simulink model "HelicopterLinear"  (R2023a)
settings: Solver=ode4  StartTime=0.0  StopTime=inf  FixedStep=0.1  RelTol=1e-3
values from neighbouring files (symbols this model uses):
  A_c = [0, 0, 1, 0 ... (first row only)    [init.m]
  B_c = [0, 0 ... (first row only)    [init.m]
  B_p = 0.01    [init.m]
  B_y = 0.08    [init.m]
  g = 9.81    [init.m]
  j_eq_p = 0.0172    [init.m]
  j_eq_y = 0.0210    (= 0.021)    [init.m]
  K_pp = 0.0556    [init.m]
  K_py = 0.005    [init.m]
  K_yp = 0.15    [init.m]
  K_yy = 0.21084    [init.m]
  l_cm = 0.015    [init.m]
  m_heli = 0.479    [init.m]
  psi_op = pi/2    (= 1.57079632679)    [init.m]
  teta_op = -10*pi/180    (= -0.174532925199)    [init.m]
  V_mp_op = K_yy*m_heli*g*cos(teta_op)*l_cm/(K_yy*K_pp - K_yp*K_py)    [init.m]
  v_my_op = K_yp*V_mp_op/K_yy    [init.m]
  wpsi_op = 0    [init.m]
  wteta_op = 0    [init.m]
libraries: simulink_extras x6
settings Model: Creator=Jardar Fagerlund  LastModifiedBy=Jardar Fagerlund

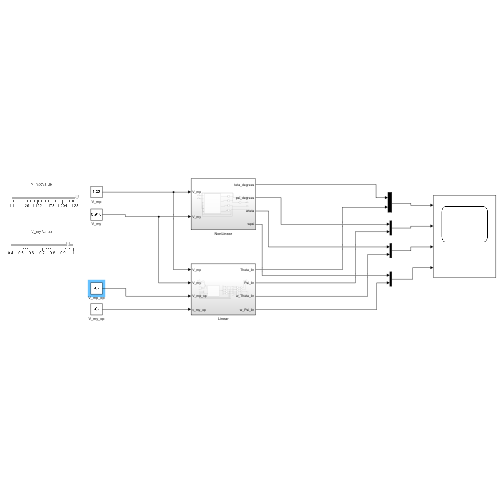
[thumbnail: Simulink's stored preview of the top-level diagram]
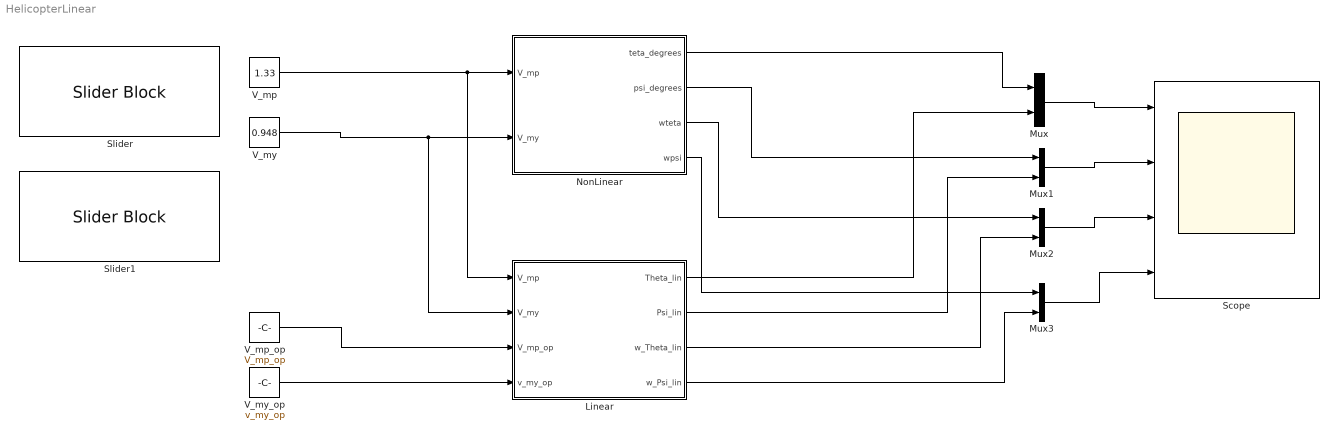
== system HelicopterLinear ==
  Linear : Subsystem
  Mux{,1..3} (4 alike) : Mux  Inputs=2
  NonLinear : Subsystem
  Scope : Scope  NumInputPorts=4
  Slider : SliderBlock  ScaleMin=1.1  ScaleMax=1.23
  Slider1 : SliderBlock  ScaleMin=0.4  ScaleMax=1
  V_mp : Constant  Value=1.33
  V_mp_op : Constant  Value=V_mp_op
  V_my : Constant  Value=0.948
  V_my_op : Constant  Value=v_my_op
  wires:
  V_mp/1 -> Linear/1(V_mp), NonLinear/1(V_mp)
  V_my/1 -> Linear/2(V_my), NonLinear/2(V_my)
  NonLinear/1(teta_degrees) -> Mux/1
  NonLinear/2(psi_degrees) -> Mux1/1
  Linear/1(Theta_lin) -> Mux/2
  Linear/2(Psi_lin) -> Mux1/2
  Mux/1 -> Scope/1
  Mux1/1 -> Scope/2
  Mux2/1 -> Scope/3
  Mux3/1 -> Scope/4
  NonLinear/3(wteta) -> Mux2/1
  Linear/3(w_Theta_lin) -> Mux2/2
  NonLinear/4(wpsi) -> Mux3/1
  Linear/4(w_Psi_lin) -> Mux3/2
  V_mp_op/1 -> Linear/3(V_mp_op)
  V_my_op/1 -> Linear/4(v_my_op)

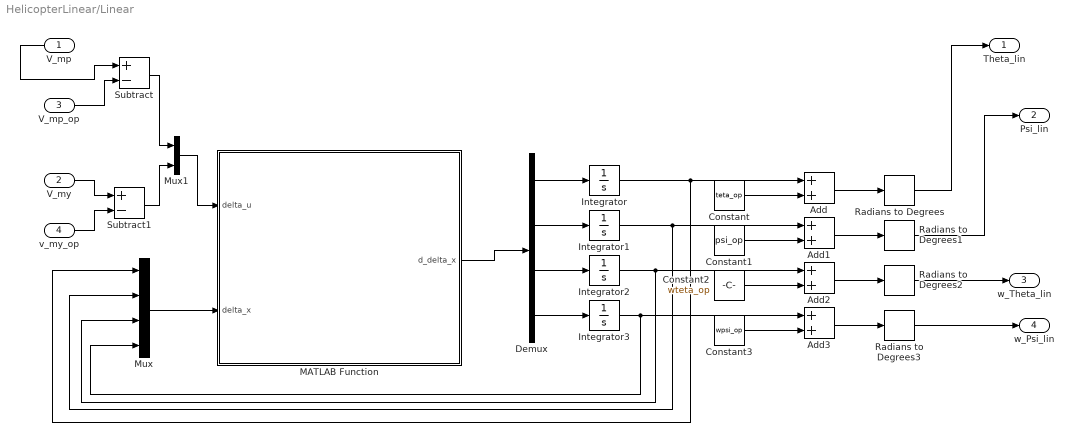
== system HelicopterLinear/Linear ==
  V_mp : Inport
  V_my : Inport  Port=2
  V_mp_op : Inport  Port=3
  v_my_op : Inport  Port=4
  Add{,1..3} (4 alike) : Sum
  Constant : Constant  Value=teta_op
  Constant1 : Constant  Value=psi_op
  Constant2 : Constant  Value=wteta_op
  Constant3 : Constant  Value=wpsi_op
  Demux : Demux
  Integrator : Integrator  LimitOutput=on  UpperSaturationLimit=35*pi/180-teta_op  LowerSaturationLimit=-45*pi/180-teta_op
  Integrator1 : Integrator  LimitOutput=on  UpperSaturationLimit=pi-psi_op  LowerSaturationLimit=0-psi_op
  Integrator2 : Integrator
  Integrator3 : Integrator
  MATLAB Function : MATLAB Function  TreatAsAtomicUnit=on
  Mux : Mux
  Mux1 : Mux  Inputs=2
  Radians to Degrees{,1..3} (4 alike) : simulink_extras/Transformations/Radians to Degrees
  Subtract : Sum  Inputs=+-
  Subtract1 : Sum  Inputs=+-
  Theta_lin : Outport
  Psi_lin : Outport  Port=2
  w_Theta_lin : Outport  Port=3
  w_Psi_lin : Outport  Port=4
  wires:
  Integrator/1 -> Mux/1, Add/1
  Integrator3/1 -> Mux/4, Add3/1
  Integrator1/1 -> Mux/2, Add1/1
  Integrator2/1 -> Mux/3, Add2/1
  Demux/1 -> Integrator/1
  Radians to Degrees1/1 -> Psi_lin/1
  Constant/1 -> Add/2
  Add2/1 -> Radians to Degrees2/1
  Demux/3 -> Integrator2/1
  Demux/4 -> Integrator3/1
  Demux/2 -> Integrator1/1
  Radians to Degrees2/1 -> w_Theta_lin/1
  MATLAB Function/1(d_delta_x) -> Demux/1
  Add3/1 -> Radians to Degrees3/1
  Constant3/1 -> Add3/2
  Constant1/1 -> Add1/2
  Constant2/1 -> Add2/2
  Add/1 -> Radians to Degrees/1
  Add1/1 -> Radians to Degrees1/1
  Radians to Degrees3/1 -> w_Psi_lin/1
  Radians to Degrees/1 -> Theta_lin/1
  V_mp/1 -> Subtract/1
  V_mp_op/1 -> Subtract/2
  V_my/1 -> Subtract1/1
  v_my_op/1 -> Subtract1/2
  Subtract1/1 -> Mux1/2
  Subtract/1 -> Mux1/1
  Mux/1 -> MATLAB Function/2(delta_x)
  Mux1/1 -> MATLAB Function/1(delta_u)

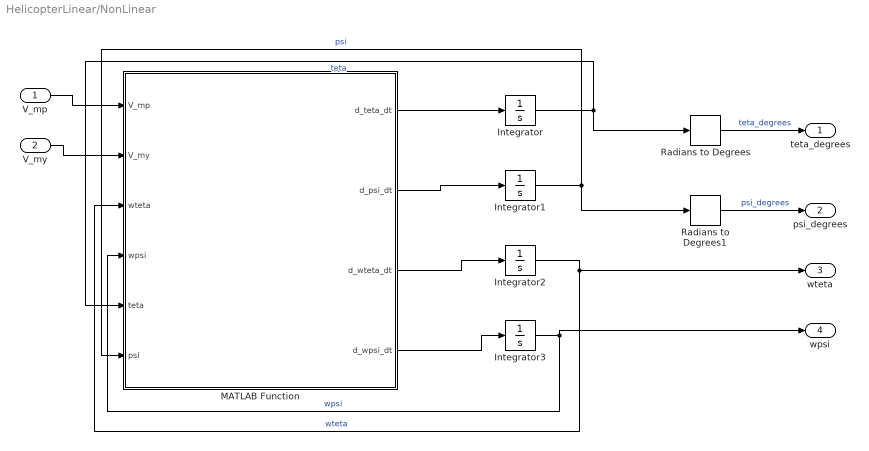
== system HelicopterLinear/NonLinear ==
  V_mp : Inport
  V_my : Inport  Port=2
  Integrator : Integrator  InitialCondition=teta_op  LimitOutput=on  UpperSaturationLimit=35*pi/180  LowerSaturationLimit=-45*pi/180
  Integrator1 : Integrator  InitialCondition=psi_op  LimitOutput=on  UpperSaturationLimit=pi  LowerSaturationLimit=0
  Integrator2 : Integrator  InitialCondition=wteta_op
  Integrator3 : Integrator  InitialCondition=wpsi_op
  MATLAB Function : MATLAB Function  TreatAsAtomicUnit=on
  Radians to Degrees : simulink_extras/Transformations/Radians to Degrees
  Radians to Degrees1 : simulink_extras/Transformations/Radians to Degrees
  teta_degrees : Outport
  psi_degrees : Outport  Port=2
  wteta : Outport  Port=3
  wpsi : Outport  Port=4
  wires:
  Integrator/1 -> Radians to Degrees/1, MATLAB Function/5(teta)  "teta"
  MATLAB Function/3(d_wteta_dt) -> Integrator2/1
  MATLAB Function/1(d_teta_dt) -> Integrator/1
  Integrator1/1 -> Radians to Degrees1/1, MATLAB Function/6(psi)  "psi"
  MATLAB Function/4(d_wpsi_dt) -> Integrator3/1
  Integrator2/1 -> wteta/1, MATLAB Function/3(wteta)  "wteta"
  V_mp/1 -> MATLAB Function/1(V_mp)
  MATLAB Function/2(d_psi_dt) -> Integrator1/1
  Integrator3/1 -> wpsi/1, MATLAB Function/4(wpsi)  "wpsi"
  Radians to Degrees/1 -> teta_degrees/1  "teta_degrees"
  Radians to Degrees1/1 -> psi_degrees/1  "psi_degrees"
  V_my/1 -> MATLAB Function/2(V_my)

== matlab function HelicopterLinear/Linear/MATLAB Function ==
  data: delta_u input; d_delta_x output; delta_x input; A_c parameter; B_c parameter; V_mp_op parameter; v_my_op parameter; teta_op parameter; psi_op parameter; wteta_op parameter; wpsi_op parameter
function d_delta_x  = HelicopterModelSimLinear(delta_u, delta_x, A_c, B_c, V_mp_op, v_my_op, teta_op, psi_op, wteta_op, wpsi_op)


d_delta_x = A_c*delta_x + B_c*delta_u;

== matlab function HelicopterLinear/NonLinear/MATLAB Function ==
  data: V_mp input; d_teta_dt output; V_my input; wteta input; wpsi input; teta input; psi input; d_psi_dt output; d_wteta_dt output; d_wpsi_dt output; K_pp parameter; K_yy parameter; l_cm parameter; m_heli parameter; j_eq_p parameter; j_eq_y parameter; g parameter; K_py parameter; K_yp parameter; B_p parameter; B_y parameter
function [d_teta_dt, d_psi_dt, d_wteta_dt, d_wpsi_dt] = HelicopterSimNonLinear(V_mp, V_my, wteta, wpsi, teta, psi, K_pp,K_yy,l_cm, m_heli, j_eq_p, j_eq_y, g, K_py, K_yp, B_p, B_y)

d_teta_dt = wteta;
d_psi_dt = wpsi;
d_wteta_dt = K_pp*V_mp/(j_eq_p + m_heli*l_cm^2) - K_py*V_my/(j_eq_p + m_heli*l_cm^2) - (B_p*wteta + m_heli*wpsi^2*sin(teta)*l_cm^2*cos(teta)+ m_heli*g*cos(teta)*l_cm)/(j_eq_p + m_heli*l_cm^2);
d_wpsi_dt = K_yp*V_mp/(j_eq_y + m_heli*cos(teta)^2*l_cm^2) - K_yy*V_my/(j_eq_y + m_heli*cos(teta)^2*l_cm^2) + 2*m_heli*wpsi*sin(teta)*l_cm^2*cos(teta)*wteta/(j_eq_y + m_heli*cos(teta)^2*l_cm^2) - B_y*wpsi/(j_eq_y+m_heli*cos(teta)^2*l_cm^2);
